simulink library "CTRL_LO_ST1_YAWTRQLAT"  (R2023b)
settings: Solver=VariableStepAuto  StartTime=0.0  StopTime=10.0  RelTol=1e-3
settings Model: Creator=blatak  LastModifiedBy=blatak

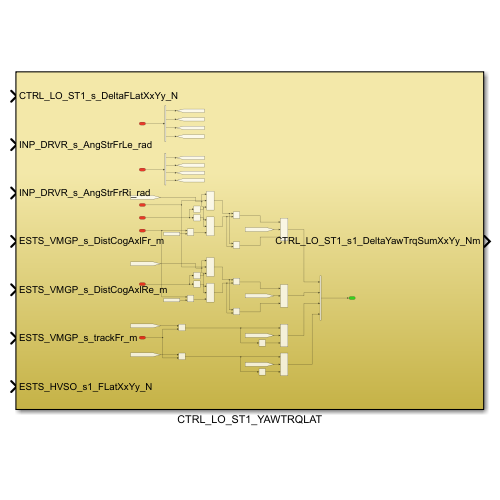
[thumbnail: Simulink's stored preview of the top-level diagram]
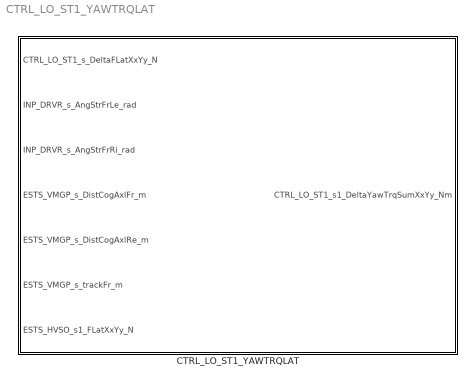
== system CTRL_LO_ST1_YAWTRQLAT ==
  CTRL_LO_ST1_YAWTRQLAT : Subsystem

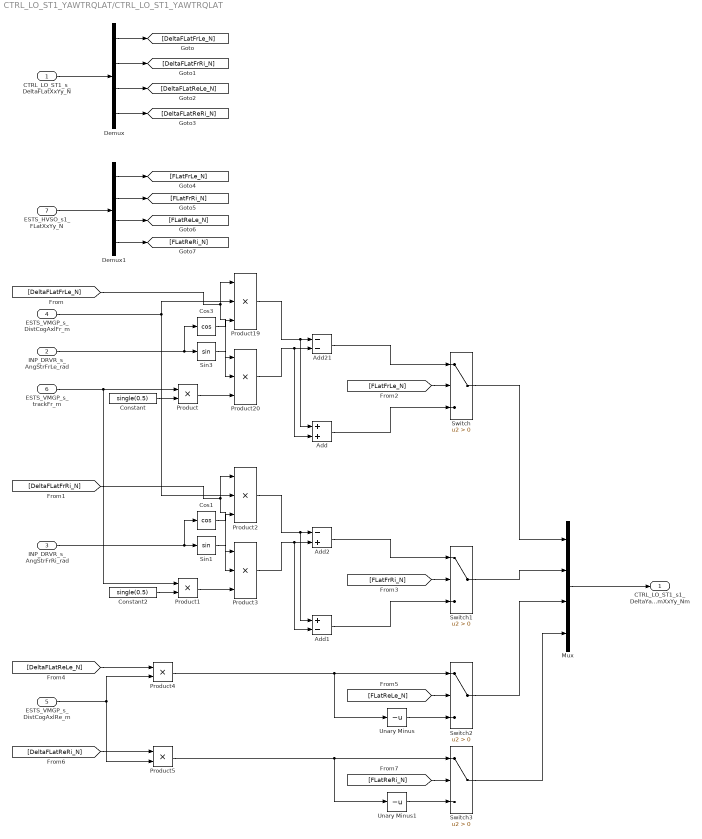
== system CTRL_LO_ST1_YAWTRQLAT/CTRL_LO_ST1_YAWTRQLAT ==
  CTRL_LO_ST1_s_DeltaFLatXxYy_N : Inport
  INP_DRVR_s_AngStrFrLe_rad : Inport  Port=2
  INP_DRVR_s_AngStrFrRi_rad : Inport  Port=3
  ESTS_VMGP_s_DistCogAxlFr_m : Inport  Port=4
  ESTS_VMGP_s_DistCogAxlRe_m : Inport  Port=5
  ESTS_VMGP_s_trackFr_m : Inport  Port=6
  ESTS_HVSO_s1_FLatXxYy_N : Inport  Port=7
  Add : Sum
  Add1 : Sum  Inputs=+-
  Add2 : Sum  Inputs=-+
  Add21 : Sum  Inputs=--
  Constant : Constant  Value=single(0.5)
  Constant2 : Constant  Value=single(0.5)
  Cos1 : Trigonometry  Operator=cos
  Cos3 : Trigonometry  Operator=cos
  Demux : Demux
  Demux1 : Demux
  Mux : Mux
  Product{,1,4..5} (4 alike) : Product
  Product{2..3,19..20} (4 alike) : Product  Inputs=3
  Sin1 : Trigonometry
  Sin3 : Trigonometry
  Switch{,1..3} (4 alike) : Switch  Criteria=u2 > Threshold  SaturateOnIntegerOverflow=off  InputSameDT=off
  Unary Minus : UnaryMinus
  Unary Minus1 : UnaryMinus
  CTRL_LO_ST1_s1_DeltaYawTrqSumXxYy_Nm : Outport
  wires:
  Product5/1 -> Unary Minus1/1, Switch3/1
  Product3/1 -> Add1/2, Add2/2
  Demux1/2 -> [FLatFrRi_N]
  Mux/1 -> CTRL_LO_ST1_s1_DeltaYawTrqSumXxYy_Nm/1
  Cos1/1 -> Product2/3
  ESTS_VMGP_s_trackFr_m/1 -> Product1/1, Product/1
  [DeltaFLatFrRi_N] -> Product2/1, Product3/1
  ESTS_HVSO_s1_FLatXxYy_N/1 -> Demux1/1
  ESTS_VMGP_s_DistCogAxlFr_m/1 -> Product19/2, Product2/2
  [FLatReLe_N] -> Switch2/2
  Product20/1 -> Add/2, Add21/2
  Product4/1 -> Unary Minus/1, Switch2/1
  Demux/1 -> [DeltaFLatFrLe_N]
  Add1/1 -> Switch1/3
  Switch/1 -> Mux/1
  INP_DRVR_s_AngStrFrLe_rad/1 -> Cos3/1, Sin3/1
  Sin1/1 -> Product3/2
  Demux/4 -> [DeltaFLatReRi_N]
  [DeltaFLatReLe_N] -> Product4/1
  [FLatReRi_N] -> Switch3/2
  ESTS_VMGP_s_DistCogAxlRe_m/1 -> Product5/2, Product4/2
  Add21/1 -> Switch/1
  Product19/1 -> Add/1, Add21/1
  [DeltaFLatFrLe_N] -> Product19/1, Product20/1
  Product1/1 -> Product3/3
  Add2/1 -> Switch1/1
  Switch3/1 -> Mux/4
  Sin3/1 -> Product20/2
  Demux/3 -> [DeltaFLatReLe_N]
  Cos3/1 -> Product19/3
  Constant2/1 -> Product1/2
  [FLatFrLe_N] -> Switch/2
  Demux1/1 -> [FLatFrLe_N]
  Demux1/4 -> [FLatReRi_N]
  INP_DRVR_s_AngStrFrRi_rad/1 -> Cos1/1, Sin1/1
  Demux/2 -> [DeltaFLatFrRi_N]
  Product2/1 -> Add1/1, Add2/1
  [FLatFrRi_N] -> Switch1/2
  Unary Minus1/1 -> Switch3/3
  Unary Minus/1 -> Switch2/3
  [DeltaFLatReRi_N] -> Product5/1
  Switch1/1 -> Mux/2
  Constant/1 -> Product/2
  Product/1 -> Product20/3
  Switch2/1 -> Mux/3
  Add/1 -> Switch/3
  Demux1/3 -> [FLatReLe_N]
  CTRL_LO_ST1_s_DeltaFLatXxYy_N/1 -> Demux/1
